simulink model "Regulador_continuo_plantilla"  (R2016a)
settings: Solver=VariableStepAuto  StartTime=0.0  StopTime=10.0  RelTol=1e-3
values from neighbouring files (symbols this model uses):
  A = [-1,0;0,2]    [Regulador_seguidor_observador_codigo.m]
  B = [1;1]    [Regulador_seguidor_observador_codigo.m]
  C = [1,1]    [Regulador_seguidor_observador_codigo.m]
  D = [0]    [Regulador_seguidor_observador_codigo.m]
  k = place(A_dis,B_dis,Pol_des_dis)    [Regulador_seguidor_observador_codigo.m]
settings Model: Creator=Daniel  LastModifiedBy=Daniel

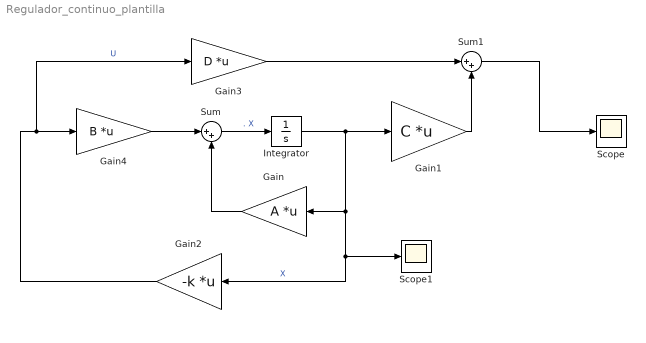
== system Regulador_continuo_plantilla ==
  Gain : Gain  Gain=A  Multiplication=Matrix(K*u) (u vector)
  Gain1 : Gain  Gain=C  Multiplication=Matrix(K*u) (u vector)
  Gain2 : Gain  Gain=-k  Multiplication=Matrix(K*u) (u vector)
  Gain3 : Gain  Gain=D  Multiplication=Matrix(K*u) (u vector)
  Gain4 : Gain  Gain=B  Multiplication=Matrix(K*u) (u vector)
  Integrator : Integrator  InitialCondition=[1;1]
  Scope : Scope
  Scope1 : Scope
  Sum : Sum  Inputs=|++
  Sum1 : Sum  Inputs=|++
  wires:
  Sum/1 -> Integrator/1  ". X"
  Gain4/1 -> Sum/1
  Gain/1 -> Sum/2
  Integrator/1 -> Gain1/1, Scope1/1, Gain2/1, Gain/1  "X"
  Gain2/1 -> Gain3/1, Gain4/1  "U"
  Sum1/1 -> Scope/1
  Gain3/1 -> Sum1/1
  Gain1/1 -> Sum1/2
